simulink model "week2_problem1"  (R2020b)
settings: Solver=VariableStepAuto  StartTime=0.0  StopTime=10.0  RelTol=1e-3
settings Model: Creator=gokul  LastModifiedBy=gokul

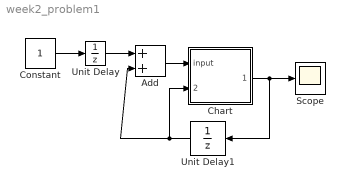
== system week2_problem1 ==
  Add : Sum
  Chart : Stateflow chart  TreatAsAtomicUnit=on
  Constant : Constant
  Scope : Scope
  Unit Delay : UnitDelay  SampleTime=-1  HasFrameUpgradeWarning=on
  Unit Delay1 : UnitDelay  SampleTime=-1  HasFrameUpgradeWarning=on
  wires:
  Add/1 -> Chart/1(input)
  Constant/1 -> Unit Delay/1
  Unit Delay/1 -> Add/1
  Unit Delay1/1 -> Chart/2(feedback), Add/2
  Chart/1(output) -> Unit Delay1/1, Scope/1

== stateflow chart week2_problem1/Chart ==
  (default) -> (junction 1) : %switch
  (junction 1) -> (junction 3) [order 2] : [feedback>=5]
  (junction 1) -> (junction 5) [order 1] : {output=input;}
  (junction 3) -> (junction 4) : {output=0;}
  (junction 4) -> (junction 5)
  (junction 5) -> (junction 6)
  data: input input; feedback input; output output
